simulink model "SF009A_DutyCycThermProtn"  (R2013b)
settings: Solver=FixedStepDiscrete  SolverMode=SingleTasking  StartTime=0.0  StopTime=1  FixedStep=0.1  RelTol=1e-3
values from neighbouring files (symbols this model uses):
  AbsltTThermLimCnt = DataDict.NTC    [SF009A_DutyCycThermProtn_DataDict.m]
  ARCHGLBPRM_100MILLISEC_SEC_F32 = DataDict.Constant    [SF009A_DutyCycThermProtn_DataDict.m]
  CTRLRANDCUTFLT_CNT_U08 = DataDict.Constant    [SF009A_DutyCycThermProtn_DataDict.m]
  CTRLRTFLT_CNT_U08 = DataDict.Constant    [SF009A_DutyCycThermProtn_DataDict.m]
  CUTFLT_CNT_U08 = DataDict.Constant    [SF009A_DutyCycThermProtn_DataDict.m]
  DITHERMLIM_MOTNWTMTR_F32 = DataDict.Constant    [SF009A_DutyCycThermProtn_DataDict.m]
  DutyCycExcddCnt = DataDict.NTC    [SF009A_DutyCycThermProtn_DataDict.m]
  DutyCycThermProtnAbsltCtrlTTblX = DataDict.Calibration    [SF009A_DutyCycThermProtn_DataDict.m]
  DutyCycThermProtnAbsltCtrlTTqTblY = DataDict.Calibration    [SF009A_DutyCycThermProtn_DataDict.m]
  DutyCycThermProtnAbsltCuTTblX = DataDict.Calibration    [SF009A_DutyCycThermProtn_DataDict.m]
  DutyCycThermProtnAbsltCuTTqTblY = DataDict.Calibration    [SF009A_DutyCycThermProtn_DataDict.m]
  DutyCycThermProtnAbsltMotVelBreakPt = DataDict.Calibration    [SF009A_DutyCycThermProtn_DataDict.m]
  DutyCycThermProtnAbsltTTqSlewHiLim = DataDict.Calibration    [SF009A_DutyCycThermProtn_DataDict.m]
  DutyCycThermProtnAbsltTTqSlewLoLim = DataDict.Calibration    [SF009A_DutyCycThermProtn_DataDict.m]
  DutyCycThermProtnCtrlT = DataDict.Calibration    [SF009A_DutyCycThermProtn_DataDict.m]
  DutyCycThermProtnCtrlTSeln = DataDict.Calibration    [SF009A_DutyCycThermProtn_DataDict.m]
  DutyCycThermProtnDutyCycFildThd = DataDict.Calibration    [SF009A_DutyCycThermProtn_DataDict.m]
  DutyCycThermProtnIgnOffCtrlEna = DataDict.Calibration    [SF009A_DutyCycThermProtn_DataDict.m]
  DutyCycThermProtnIgnOffMsgWaitTi = DataDict.Calibration    [SF009A_DutyCycThermProtn_DataDict.m]
  DutyCycThermProtnLstTblValNonStall = DataDict.Calibration    [SF009A_DutyCycThermProtn_DataDict.m]
  DutyCycThermProtnLstTblValStall = DataDict.Calibration    [SF009A_DutyCycThermProtn_DataDict.m]
  DutyCycThermProtnMotPrTSeln = DataDict.Calibration    [SF009A_DutyCycThermProtn_DataDict.m]
  DutyCycThermProtnMplr1NonStallTblY = DataDict.Calibration    [SF009A_DutyCycThermProtn_DataDict.m]
  DutyCycThermProtnMplr1StallTblY = DataDict.Calibration    [SF009A_DutyCycThermProtn_DataDict.m]
  DutyCycThermProtnMplr2NonStallTblY = DataDict.Calibration    [SF009A_DutyCycThermProtn_DataDict.m]
  DutyCycThermProtnMplr2StallTblY = DataDict.Calibration    [SF009A_DutyCycThermProtn_DataDict.m]
  DutyCycThermProtnMplr3NonStallTblY = DataDict.Calibration    [SF009A_DutyCycThermProtn_DataDict.m]
  DutyCycThermProtnMplr3StallTblY = DataDict.Calibration    [SF009A_DutyCycThermProtn_DataDict.m]
  DutyCycThermProtnMplr4NonStallTblY = DataDict.Calibration    [SF009A_DutyCycThermProtn_DataDict.m]
  DutyCycThermProtnMplr4StallTblY = DataDict.Calibration    [SF009A_DutyCycThermProtn_DataDict.m]
  DutyCycThermProtnMplr5NonStallTblY = DataDict.Calibration    [SF009A_DutyCycThermProtn_DataDict.m]
  DutyCycThermProtnMplr5StallTblY = DataDict.Calibration    [SF009A_DutyCycThermProtn_DataDict.m]
  DutyCycThermProtnMplr6NonStallTblY = DataDict.Calibration    [SF009A_DutyCycThermProtn_DataDict.m]
  DutyCycThermProtnMplr6StallTblY = DataDict.Calibration    [SF009A_DutyCycThermProtn_DataDict.m]
  DutyCycThermProtnMplrTblX = DataDict.Calibration    [SF009A_DutyCycThermProtn_DataDict.m]
  DutyCycThermProtnMplrTSeln = DataDict.Calibration    [SF009A_DutyCycThermProtn_DataDict.m]
  DutyCycThermProtnSlowFilTSeln = DataDict.Calibration    [SF009A_DutyCycThermProtn_DataDict.m]
  DutyCycThermProtnThermLimScaFac = DataDict.Calibration    [SF009A_DutyCycThermProtn_DataDict.m]
  DutyCycThermProtnThermLoadLimTblX = DataDict.Calibration    [SF009A_DutyCycThermProtn_DataDict.m]
  DutyCycThermProtnThermLoadLimTblY = DataDict.Calibration    [SF009A_DutyCycThermProtn_DataDict.m]
  DutyCycThermProtnTqCmdSlewDwn = DataDict.Calibration    [SF009A_DutyCycThermProtn_DataDict.m]
  DutyCycThermProtnTqCmdSlewUp = DataDict.Calibration    [SF009A_DutyCycThermProtn_DataDict.m]
  FILVALMIN_ULS_F32 = DataDict.Constant    [SF009A_DutyCycThermProtn_DataDict.m]
  IGNTIOFFTHD_CNT_F32 = DataDict.Constant    [SF009A_DutyCycThermProtn_DataDict.m]
  NODEBSTEP_CNT_U16 = DataDict.Constant    [SF009A_DutyCycThermProtn_DataDict.m]
  ONEPERC_ULS_F32 = DataDict.Constant    [SF009A_DutyCycThermProtn_DataDict.m]
  TAU3_SEC_F32 = DataDict.Constant    [SF009A_DutyCycThermProtn_DataDict.m]
  TAU4_SEC_F32 = DataDict.Constant    [SF009A_DutyCycThermProtn_DataDict.m]
  TAU5_SEC_F32 = DataDict.Constant    [SF009A_DutyCycThermProtn_DataDict.m]
  TAU6_SEC_F32 = DataDict.Constant    [SF009A_DutyCycThermProtn_DataDict.m]
  THERMLOADLIMTBLIDX_ULS_U08 = DataDict.Constant    [SF009A_DutyCycThermProtn_DataDict.m]
undefined symbols (not defined in the file or in its folder): NtcSts1, NvmGetErrSts1
libraries: FixdToFloat x13, Fil x12, NxtrLim x12, simulink x11, NxtrMath x8, FloatToFixd x6, NxtrMax x6, NxtrMin x3, NxtrAbslt x2, NxtrNvM x1
(part 7 of 7)

== stateflow chart SF009A_DutyCycThermProtn/DutyCycThermProtn/DutyCycThermProtnPer1/TempratureLimiting/SetNtc/SetNtcSts/ISO Fault Debounce Design ==
  note: NTCSTS_PASSD           (0)
      | NTCSTS_FAILD             (1)
      | NTCSTS_PREPASSD   (2)
      | NTCSTS_PREFAILD     (3)
      |
      | SIGQLFR_NORES        (0)
      | SIGQLFR_PASSD         (1)
      | SIGQLFR_FAILD           (2)
  note: Pass Loop
  note: Fail Loop
  note: 
  (default) -> (junction 89)
  (junction 89) -> (junction 95) [order 1] : [NtcSts ==3]
  (junction 89) -> (junction 93) [order 2] : [NtcSts ==2]
  (junction 89) -> (junction 141) [order 3] : [NtcSts ==1]
      | { ErrAcc = 200;
      | Qualifier =2;
      |  }
  (junction 89) -> (junction 141) [order 4] : [NtcSts ==0]
      | { ErrAcc = 0;
      | Qualifier=1;
      | }
  (junction 95) -> (junction 103) [order 2]
  (junction 95) -> (junction 111) [order 1] : [ErrAcc <=0]
      | {ErrAcc = DebStep;}
  (junction 93) -> (junction 123) [order 2] : {
      | ErrAcc = ErrAcc - DebStep;
      | }
  (junction 93) -> (junction 123) [order 1] : [(ErrAcc - DebStep) <= 0]
      | { ErrAcc = 0;
      | Qualifier=1;
      | }
  (junction 103) -> (junction 111) [order 1] : [(ErrAcc + DebStep) <200]
      | {ErrAcc = ErrAcc + DebStep;}
  (junction 103) -> (junction 111) [order 2] : {ErrAcc = 200;
      | Qualifier =2;}
  (junction 123) -> (junction 141)
  (junction 111) -> (junction 141)
  (junction 141) -> (junction 159) [order 2]
  (junction 141) -> (junction 159) [order 1] : [SvcClr ==0]
  data: NtcSts input Enum: NtcSts1; Qualifier output uint8; DebStep input; ErrAcc local single; SvcClr input

== stateflow chart SF009A_DutyCycThermProtn/DutyCycThermProtn/DutyCycThermProtnPer1/ThermalLimitStatus/MaxoutLimiting/SetNtcFail/SetNtcSts/ISO Fault Debounce Design ==
  note: NTCSTS_PASSD           (0)
      | NTCSTS_FAILD             (1)
      | NTCSTS_PREPASSD   (2)
      | NTCSTS_PREFAILD     (3)
      |
      | SIGQLFR_NORES        (0)
      | SIGQLFR_PASSD         (1)
      | SIGQLFR_FAILD           (2)
  note: Pass Loop
  note: Fail Loop
  note: 
  (default) -> (junction 89)
  (junction 89) -> (junction 95) [order 1] : [NtcSts ==3]
  (junction 89) -> (junction 93) [order 2] : [NtcSts ==2]
  (junction 89) -> (junction 141) [order 3] : [NtcSts ==1]
      | { ErrAcc = 200;
      | Qualifier =2;
      |  }
  (junction 89) -> (junction 141) [order 4] : [NtcSts ==0]
      | { ErrAcc = 0;
      | Qualifier=1;
      | }
  (junction 95) -> (junction 103) [order 2]
  (junction 95) -> (junction 111) [order 1] : [ErrAcc <=0]
      | {ErrAcc = DebStep;}
  (junction 93) -> (junction 123) [order 2] : {
      | ErrAcc = ErrAcc - DebStep;
      | }
  (junction 93) -> (junction 123) [order 1] : [(ErrAcc - DebStep) <= 0]
      | { ErrAcc = 0;
      | Qualifier=1;
      | }
  (junction 103) -> (junction 111) [order 1] : [(ErrAcc + DebStep) <200]
      | {ErrAcc = ErrAcc + DebStep;}
  (junction 103) -> (junction 111) [order 2] : {ErrAcc = 200;
      | Qualifier =2;}
  (junction 123) -> (junction 141)
  (junction 111) -> (junction 141)
  (junction 141) -> (junction 159) [order 2]
  (junction 141) -> (junction 159) [order 1] : [SvcClr ==0]
  data: NtcSts input Enum: NtcSts1; Qualifier output uint8; DebStep input; ErrAcc local single; SvcClr input

== stateflow chart SF009A_DutyCycThermProtn/DutyCycThermProtn/DutyCycThermProtnPer1/ThermalLimitStatus/MaxoutLimiting/SetNtcPass/SetNtcSts/ISO Fault Debounce Design ==
  note: NTCSTS_PASSD           (0)
      | NTCSTS_FAILD             (1)
      | NTCSTS_PREPASSD   (2)
      | NTCSTS_PREFAILD     (3)
      |
      | SIGQLFR_NORES        (0)
      | SIGQLFR_PASSD         (1)
      | SIGQLFR_FAILD           (2)
  note: Pass Loop
  note: Fail Loop
  note: 
  (default) -> (junction 89)
  (junction 89) -> (junction 95) [order 1] : [NtcSts ==3]
  (junction 89) -> (junction 93) [order 2] : [NtcSts ==2]
  (junction 89) -> (junction 141) [order 3] : [NtcSts ==1]
      | { ErrAcc = 200;
      | Qualifier =2;
      |  }
  (junction 89) -> (junction 141) [order 4] : [NtcSts ==0]
      | { ErrAcc = 0;
      | Qualifier=1;
      | }
  (junction 95) -> (junction 103) [order 2]
  (junction 95) -> (junction 111) [order 1] : [ErrAcc <=0]
      | {ErrAcc = DebStep;}
  (junction 93) -> (junction 123) [order 2] : {
      | ErrAcc = ErrAcc - DebStep;
      | }
  (junction 93) -> (junction 123) [order 1] : [(ErrAcc - DebStep) <= 0]
      | { ErrAcc = 0;
      | Qualifier=1;
      | }
  (junction 103) -> (junction 111) [order 1] : [(ErrAcc + DebStep) <200]
      | {ErrAcc = ErrAcc + DebStep;}
  (junction 103) -> (junction 111) [order 2] : {ErrAcc = 200;
      | Qualifier =2;}
  (junction 123) -> (junction 141)
  (junction 111) -> (junction 141)
  (junction 141) -> (junction 159) [order 2]
  (junction 141) -> (junction 159) [order 1] : [SvcClr ==0]
  data: NtcSts input Enum: NtcSts1; Qualifier output uint8; DebStep input; ErrAcc local single; SvcClr input
